simulink model "Model"  (R2024b)
settings: Solver=VariableStepAuto  StartTime=0.0  StopTime=1  RelTol=1e-3
undefined symbols (not defined in the file): D1, Delta
libraries: spsThreePhaseTransformerTwoWindingsLib x4, spsThreePhaseProgrammableVoltageSourceLib x2, spsGroundLib x2, spsDistributedParametersLineLib x2, spsThreePhaseMutualInductanceZ1Z0Lib x2, spsThreePhaseFaultLib x1, spsThreePhaseParallelRLCLoadLib x1, spsThreePhaseVIMeasurementLib x1, sps_lib x1
settings Model: Creator=SJ  LastModifiedBy=janme
settings RTWCC: GPUComputeCapability=3.5

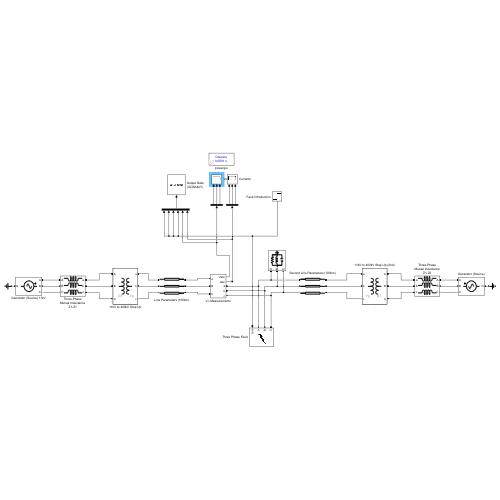
[thumbnail: Simulink's stored preview of the top-level diagram]
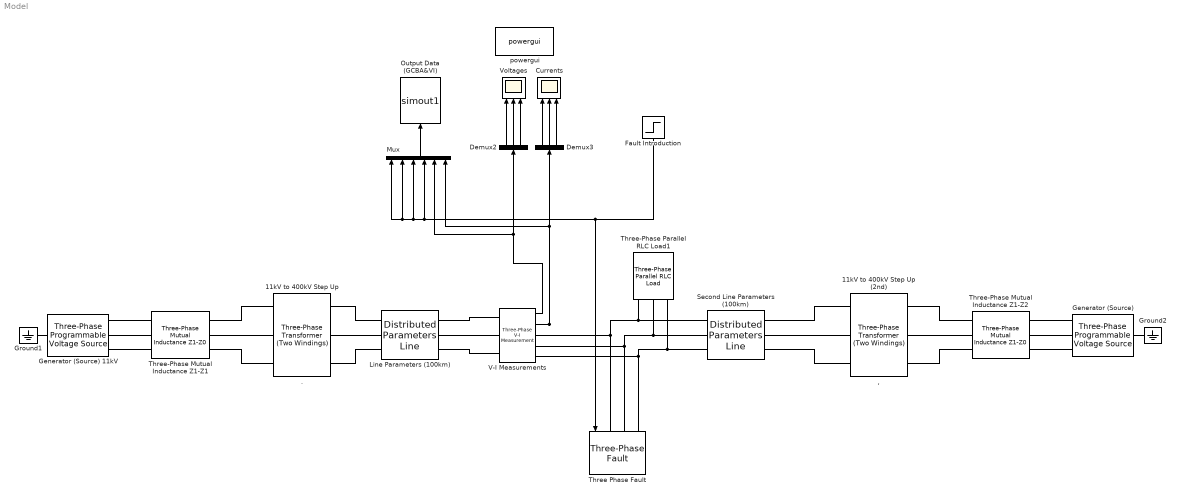
== system Model ==
  , : spsThreePhaseTransformerTwoWindingsLib/Three-Phase Transformer (Two Windings)  Winding1Connection=Delta (D1)  Winding2Connection=Yg  CoreType=Three single-phase transformers  SetSaturation=off  Hysteresis=off  DataFile='hysteresis'  SetInitialFlux=off  Measurements=None  UNITS=pu  NominalPower=[ 2500e3 , 50 ]  Winding1=[ 11e3 , 0.002 , 0.08 ]  Winding2=[ 4e5, 0.002, 0.08 ]  Rm=500  Lm=500  L0=0.5  Saturation=[ 0,0 ; 0.0024,1.2 ; 1.0,1.52 ]  InitialFluxes=[ 0.8 , -0.8 , 0.7 ]  BreakLoop=off  DiscreteSolver=Trapezoidal iterative  DataType=off  TransfoNumber=1
  . : spsThreePhaseTransformerTwoWindingsLib/Three-Phase Transformer (Two Windings)  Winding1Connection=Delta (D1)  Winding2Connection=Yg  CoreType=Three single-phase transformers  SetSaturation=off  Hysteresis=off  DataFile='hysteresis'  SetInitialFlux=off  Measurements=None  UNITS=pu  NominalPower=[ 2500e3 , 50 ]  Winding1=[ 11e3 , 0.002 , 0.08 ]  Winding2=[ 4e5, 0.002, 0.08 ]  Rm=500  Lm=500  L0=0.5  Saturation=[ 0,0 ; 0.0024,1.2 ; 1.0,1.52 ]  InitialFluxes=[ 0.8 , -0.8 , 0.7 ]  BreakLoop=off  DiscreteSolver=Trapezoidal iterative  DataType=off  TransfoNumber=1
  11kV to 400kV Step Up : spsThreePhaseTransformerTwoWindingsLib/Three-Phase Transformer (Two Windings)  Winding1Connection=Delta (D1)  Winding2Connection=Yg  CoreType=Three single-phase transformers  SetSaturation=off  Hysteresis=off  DataFile='hysteresis'  SetInitialFlux=off  Measurements=None  UNITS=pu  NominalPower=[ 2500e3 , 50 ]  Winding1=[ 11e3 , 0.002 , 0.08 ]  Winding2=[ 4e2, 0.002, 0.08 ]  Rm=500  Lm=500  L0=0.5  Saturation=[ 0,0 ; 0.0024,1.2 ; 1.0,1.52 ]  InitialFluxes=[ 0.8 , -0.8 , 0.7 ]  BreakLoop=off  DiscreteSolver=Trapezoidal iterative  DataType=off  TransfoNumber=1
  11kV to 400kV Step Up (2nd) : spsThreePhaseTransformerTwoWindingsLib/Three-Phase Transformer (Two Windings)  Winding1Connection=Delta (D1)  Winding2Connection=Yg  CoreType=Three single-phase transformers  SetSaturation=off  Hysteresis=off  DataFile='hysteresis'  SetInitialFlux=off  Measurements=None  UNITS=pu  NominalPower=[ 2500e3 , 50 ]  Winding1=[ 11e3 , 0.002 , 0.08 ]  Winding2=[ 4e2 , 0.002 , 0.08 ]  Rm=500  Lm=500  L0=0.5  Saturation=[ 0,0 ; 0.0024,1.2 ; 1.0,1.52 ]  InitialFluxes=[ 0.8 , -0.8 , 0.7 ]  BreakLoop=off  DiscreteSolver=Trapezoidal iterative  DataType=off  TransfoNumber=1
  Currents : Scope  NumInputPorts=3
  Demux2 : Demux  Outputs=3
  Demux3 : Demux  Outputs=3
  Fault Introduction : Step  Time=0.1  SampleTime=0
  Generator (Source) : spsThreePhaseProgrammableVoltageSourceLib/Three-Phase Programmable Voltage Source  PositiveSequence="[11e3  0 50]"  VariationEntity=None  VariationType=Table of time-amplitude pairs  VariationTypeAlt=Step  VariationStep=0.5  VariationRate=10  VariationMagnitude=0.3  VariationFrequency=2  VariationTiming=[1 2]  VariationPhaseA=off  Amplitudes=[1 0.8 1.2 1.0]  TimeValues=[0 0.1 0.15 0.2]  HarmonicGeneration=off  HarmonicA=[3 0.2 -25 0]  HarmonicB=[2 0.15 35 2]  Timing="[0.05  3]"  BusType=swing  Pref=0  Qref=0  Qmin=-inf  Qmax=inf
  Generator (Source) 11kV : spsThreePhaseProgrammableVoltageSourceLib/Three-Phase Programmable Voltage Source  PositiveSequence="[11e3  0 50]"  VariationEntity=None  VariationType=Table of time-amplitude pairs  VariationTypeAlt=Step  VariationStep=0.5  VariationRate=10  VariationMagnitude=0.3  VariationFrequency=2  VariationTiming=[1 2]  VariationPhaseA=off  Amplitudes=[1 0.8 1.2 1.0]  TimeValues=[0 0.1 0.15 0.2]  HarmonicGeneration=off  HarmonicA=[3 0.2 -25 0]  HarmonicB=[2 0.15 35 2]  Timing="[0.05  3]"  BusType=swing  Pref=0  Qref=0  Qmin=-inf  Qmax=inf
  Ground1 : spsGroundLib/Ground  LConnTagsString=a
  Ground2 : spsGroundLib/Ground  LConnTagsString=a
  Line Parameters (100km) : spsDistributedParametersLineLib/Distributed Parameters Line  Phases=3  Length=100  Frequency=50  Resistance=[0.01273 0.3864]  Inductance="[0.9337e-3  4.1264e-3]"  Capacitance=[12.74e-9 7.751e-9]  x1=[-0.0006 3.5059065032272e-14 302.29132914741 -261.391829825195;-0.0005 3.87975771982441e-14 310.352682416144 -251.767648625028;-0.0004 4.24978008396097e-14 318.107755056666 -241.895003151946;-0.0003 4.61560842823684e-14 325.548893748561 -231.78363651509;-0.0002 4.97688172424319e-14 332.668754986322 -221.443527412571;-0.0001 5.33324343885393e-14 339.460312326496 -210.884880283698]  x2=[-0.0006 -1.95427979721808e-13 258.197390789364 -298.948014119863;-0.0005 -1.9650253716935e-13 267.460170011688 -290.690325284424;-0.0004 -1.97383170336745e-13 276.458998337068 -282.145760193398;-0.0003 -1.98069010145376e-13 285.184995008388 -273.322751300931;-0.0002 -1.98559379754155e-13 293.629548520437 -264.230005851587;-0.0001 -1.98853795227482e-13 301.784325118422 -254.876497287341]  x3=[-0.0006 9.51421072081164e-16 -0.281911370788044 0.421950096006031;-0.0005 8.84911361054694e-16 -0.295026037352985 0.41288683895577;-0.0004 8.17528349351507e-16 -0.307849548837983 0.403416112443892;-0.0003 7.49338535868903e-16 -0.320369249985404 0.39354726293405;-0.0002 6.80409215720135e-16 -0.332572785361739 0.383290029789228;-0.0001 6.10808413822251e-16 -0.34444811155092 0.37265453566017]  x4=[-0.0006 -1.59862770096895e-15 2.23300549703812 -2.5964882734215;-0.0005 -1.5520993023876e-15 2.31346131122797 -2.52506666550988;-0.0004 -1.50403916918202e-15 2.39163401841121 -2.45115312165439;-0.0003 -1.45449473090131e-15 2.46744647156375 -2.37482058559914;-0.0002 -1.40351488192447e-15 2.54082385294728 -2.29614438834146;-0.0001 -1.35114993320758e-15 2.61169374794533 -2.21520217378936]  x5=0.000565541566995743  V1=[2.024e-13 399.6 399.6;314.2 314.2 314.2;-1.932 0.938 -0.6328]  V2=[2.05e-13 395 395;314.2 314.2 314.2;0.8051 0.7925 -0.7783]  I1=[3.039e-15 0.5075 0.5075;314.2 314.2 314.2;-0.08862 -2.472 2.24]  I2=[2.819e-15 3.425 3.425;314.2 314.2 314.2;3.041 0.7904 -0.7804]  nHarmo=1  Measurements=None  Decoupling=off  VsMag0=0  VrMag0=0  VsAngle0=0  VrAngle0=0  IsMag0=0  IrMag0=0  IsAngle0=0  IrAngle0=0
      settings: LibrarySourceBlock=sps_lib/Power Grid Elements/Distributed Parameters Line
  Mux : Mux  Inputs=6
  Output Data (GCBA&VI) : ToWorkspace  VariableName=simout1  SaveFormat=Timeseries  SampleTime=-1
  Second Line Parameters (100km) : spsDistributedParametersLineLib/Distributed Parameters Line  Phases=3  Length=100  Frequency=60  Resistance=[0.01273 0.3864]  Inductance="[0.9337e-3  4.1264e-3]"  Capacitance=[12.74e-9 7.751e-9]  x1=[-0.0006 -2.54114646410191e-13 302.291329147411 -261.391829825195;-0.0005 -2.50261177929072e-13 310.352682416144 -251.767648625029;-0.0004 -2.46160731879736e-13 318.107755056666 -241.895003151946;-0.0003 -2.4181735490738e-13 325.548893748562 -231.78363651509;-0.0002 -2.37235333400693e-13 332.668754986322 -221.443527412572;-0.0001 -2.32419189261709e-13 339.460312326496 -210.884880283698]  x2=[-0.0006 -1.95427979721808e-13 258.197390789364 -298.948014119863;-0.0005 -1.9650253716935e-13 267.460170011688 -290.690325284424;-0.0004 -1.97383170336745e-13 276.458998337068 -282.145760193398;-0.0003 -1.98069010145376e-13 285.184995008388 -273.322751300931;-0.0002 -1.98559379754155e-13 293.629548520437 -264.230005851587;-0.0001 -1.98853795227482e-13 301.784325118422 -254.876497287341]  x3=[-0.0006 -2.40981597033805e-17 -0.28191137078804 0.421950096006025;-0.0005 -1.55871589637802e-17 -0.295026037352981 0.412886838955764;-0.0004 -7.06077558014317e-18 -0.30784954883798 0.403416112443886;-0.0003 1.4725759365337e-18 -0.320369249985401 0.393547262934043;-0.0002 1.00044741985475e-17 -0.332572785361736 0.383290029789222;-0.0001 1.85264992523821e-17 -0.344448111550917 0.372654535660164]  x4=[-0.0006 -1.27447012841234e-15 2.23300549703812 -2.5964882734215;-0.0005 -1.28147778089948e-15 2.31346131122797 -2.52506666550988;-0.0004 -1.28722076953157e-15 2.39163401841121 -2.45115312165439;-0.0003 -1.29169342667217e-15 2.46744647156375 -2.37482058559914;-0.0002 -1.29489133834869e-15 2.54082385294728 -2.29614438834146;-0.0001 -1.29681134860838e-15 2.61169374794533 -2.21520217378936]  x5=0.000565541566995742  V1=[3.558e-13 399.6 399.6;314.2 314.2 314.2;-1.251 0.938 -0.6328]  V2=[2.05e-13 395 395;314.2 314.2 314.2;0.8051 0.7925 -0.7783]  I1=[4.38e-15 0.5075 0.5075;314.2 314.2 314.2;0.2418 -2.472 2.24]  I2=[2.604e-15 3.425 3.425;314.2 314.2 314.2;-2.475 0.7904 -0.7804]  nHarmo=1  Measurements=None  Decoupling=off  VsMag0=0  VrMag0=0  VsAngle0=0  VrAngle0=0  IsMag0=0  IrMag0=0  IsAngle0=0  IrAngle0=0
      settings: LibrarySourceBlock=sps_lib/Power Grid Elements/Distributed Parameters Line
  Three Phase Fault : spsThreePhaseFaultLib/Three-Phase Fault  InitialStates=0  FaultA=on  FaultB=on  FaultC=on  GroundFault=on  SwitchTimes=[0.25]  External=on  SwitchStatus=NaN  FaultResistance=0.001  GroundResistance=0.01  SnubberResistance=1e6  SnubberCapacitance=inf  Measurements=None
  Three-Phase Mutual Inductance Z1-Z1 : spsThreePhaseMutualInductanceZ1Z0Lib/Three-Phase Mutual Inductance Z1-Z0  LConnTagsString=a|b|c  RConnTagsString=A|B|C  PositiveSequence="[ 2  50e-3]"  ZeroSequence="[4  100e-3]"
      settings: AttributesFormatString=\n
      settings: LibrarySourceBlock=|
      | sps_lib/Power Grid Elements/Three-Phase
      | Mutual Inductance
      | Z1-Z0
  Three-Phase Mutual Inductance Z1-Z2 : spsThreePhaseMutualInductanceZ1Z0Lib/Three-Phase Mutual Inductance Z1-Z0  LConnTagsString=a|b|c  RConnTagsString=A|B|C  PositiveSequence="[ 2  50e-3]"  ZeroSequence="[4  100e-3]"
      settings: AttributesFormatString=\n
      settings: LibrarySourceBlock=|
      | sps_lib/Power Grid Elements/Three-Phase
      | Mutual Inductance
      | Z1-Z0
  Three-Phase Parallel RLC Load1 : spsThreePhaseParallelRLCLoadLib/Three-Phase Parallel RLC Load  LConnTagsString=A|B|C  Configuration=Y (grounded)  NominalVoltage=1000  Vabc=[1e3 1e3 1e3]  Vabcp=[1e3 1e3 1e3]  NominalFrequency=60  UnbalancedPower=off  ActivePower=10e3  InductivePower=100  CapacitivePower=100  Pabc=[10e3 9e3 11e3]  QLabc=[100 90 110]  QCabc=[100 90 110]  Pabcp=[10e3 9e3 11e3]  QLabcp=[100 90 110]  QCabcp=[100 90 110]  Measurements=None  LoadType=constant Z
  V-I Measurements : spsThreePhaseVIMeasurementLib/Three-Phase V-I Measurement  VoltageMeasurement=phase-to-phase  SetLabelV=off  LabelV=Vabc  Vpu=off  VpuLL=off  CurrentMeasurement=yes  SetLabelI=off  LabelI=Iabc  Ipu=off  Pbase=2500e6  Vbase=400  OutputType=Complex  PhasorSimulation=off  PSBequivalent=0
  Voltages : Scope  NumInputPorts=3
  powergui : sps_lib/powergui  Priority=1  SimulationMode=Discrete  SampleTime=1e-4  frequency=60  Iterations=50  frequencyindice=50  Pbase=100e6  ErrMax=1e-4  UnitsV=kV  UnitsW=MW  buscounter=0  FunctionMessages=off  echomessages=off  EnableUseOfTLC=off  CurrentSourceSwitches=off  DisableSnubberDevices=off  DisableRonSwitches=off  DisableVfSwitches=off  DisplayEquations=off  AutomaticDiscreteSolvers=off  SolverType=Tustin/Backward Euler (TBE)  Interpol=off  ExternalGateDelay=off  methode=off  Ts=100  x0status=blocks  SPID=on  SwTol=0  HookPort=off  NonlinearTolerance=1e-4  nMaxIteration=100  ContinueOnMaxIteration=off  RestoreLinks=warning  ResistiveCurrentMeasurement=off  Frange=[0:2:500]  Ylog=off  Xlog=on  ShowGrid=off  save=off  variable=ZData  structure=0  ZoomFFT=off  StartTime=0.0  cycles=1  DisplayStyle=1  fundamental=60  FreqAxis=off  MaxFrequency=1000  frequencyindicesteady=1  RmsSteady=1  display=off
  wires:
  Demux3/2 -> Currents/2
  Demux3/1 -> Currents/1
  Demux2/1 -> Voltages/1
  Demux3/3 -> Currents/3
  Demux2/2 -> Voltages/2
  Demux2/3 -> Voltages/3
  V-I Measurements/2 -> Mux/6, Demux3/1
  V-I Measurements/1 -> Mux/5, Demux2/1
  Fault Introduction/1 -> Three Phase Fault/1, Mux/4, Mux/3, Mux/1, Mux/2
  Mux/1 -> Output Data (GCBA&VI)/1
  connections:
  V-I Measurements/RConn3 -- Second Line Parameters (100km)/RConn3 -- Three-Phase Parallel RLC Load1/LConn3 -- Three Phase Fault/LConn3
  Second Line Parameters (100km)/RConn2 -- V-I Measurements/RConn2 -- Three Phase Fault/LConn2 -- Three-Phase Parallel RLC Load1/LConn2
  Second Line Parameters (100km)/RConn1 -- V-I Measurements/RConn1 -- Three Phase Fault/LConn1 -- Three-Phase Parallel RLC Load1/LConn1
  Ground1/LConn1 -- Generator (Source) 11kV/LConn1
  Line Parameters (100km)/RConn3 -- V-I Measurements/LConn3
  Line Parameters (100km)/RConn1 -- V-I Measurements/LConn1
  11kV to 400kV Step Up/LConn3 -- Three-Phase Mutual Inductance Z1-Z1/RConn3
  11kV to 400kV Step Up/LConn2 -- Three-Phase Mutual Inductance Z1-Z1/RConn2
  11kV to 400kV Step Up/LConn1 -- Three-Phase Mutual Inductance Z1-Z1/RConn1
  Line Parameters (100km)/RConn2 -- V-I Measurements/LConn2
  Three-Phase Mutual Inductance Z1-Z1/LConn3 -- Generator (Source) 11kV/RConn3
  Generator (Source) 11kV/RConn2 -- Three-Phase Mutual Inductance Z1-Z1/LConn2
  Three-Phase Mutual Inductance Z1-Z1/LConn1 -- Generator (Source) 11kV/RConn1
  Line Parameters (100km)/LConn3 -- 11kV to 400kV Step Up/RConn3
  Line Parameters (100km)/LConn2 -- 11kV to 400kV Step Up/RConn2
  Line Parameters (100km)/LConn1 -- 11kV to 400kV Step Up/RConn1
  Three-Phase Mutual Inductance Z1-Z2/LConn1 -- Generator (Source)/RConn1
  Second Line Parameters (100km)/LConn1 -- 11kV to 400kV Step Up (2nd)/RConn1
  11kV to 400kV Step Up (2nd)/LConn1 -- Three-Phase Mutual Inductance Z1-Z2/RConn1
  Generator (Source)/RConn2 -- Three-Phase Mutual Inductance Z1-Z2/LConn2
  Ground2/LConn1 -- Generator (Source)/LConn1
  Second Line Parameters (100km)/LConn3 -- 11kV to 400kV Step Up (2nd)/RConn3
  11kV to 400kV Step Up (2nd)/LConn2 -- Three-Phase Mutual Inductance Z1-Z2/RConn2
  Second Line Parameters (100km)/LConn2 -- 11kV to 400kV Step Up (2nd)/RConn2
  11kV to 400kV Step Up (2nd)/LConn3 -- Three-Phase Mutual Inductance Z1-Z2/RConn3
  Three-Phase Mutual Inductance Z1-Z2/LConn3 -- Generator (Source)/RConn3
